simulink model "basic_cosimulation_c_1_sm_master"  (R2021b)
settings: Solver=ode4  StartTime=0.0  StopTime=inf  FixedStep=5e-05  RelTol=1e-3  EnableMultiTasking=on
PostLoadFcn:
  | %
  | % Script for validation of swtiching model design with it's respective
  | % average model.
  | %
  | % Here it is presented the design of the inverter to the 6 kW Fuel Cell
  | % model.
  | 
  | %%% Initialization %%%
  | 
  | 
  | % ------------------------------------- %
  | % ---------- Inverter Design ---------- %
  | % ------------------------------------- %
  | 
  | %%%% Nominal Parameters %%%%
  | 
  | Pnom = 50e3;                                        % Nominal Power
  | Vdc = 400;                                          % DC Voltage - Boost
  | m = 0.6;                                            % Modulation Index
  | Vnom_peak = m*Vdc/2;                                % Peak Voltage
  | Vnom_rms = Vnom_peak/sqrt(2);                       % Rms Voltage
  | FP_min = 0.9;                                       % For Reactive Power
  |                                                     % Compensation
  | Snom = Pnom/FP_min;                                 % Apparent Power
  | Irms = Pnom/(sqrt(3)*Vnom_rms);                     % Rms Curren
  | Inom_peak = Irms*sqrt(2);                           % Peak Current
  | Zbase = Vnom_peak/Inom_peak;                        % Base Impedance
  | f = 60;                                             % Nominal Frequency
  | wnom = 2*pi*60;                                     % Angular Frequency
  | 
  | % ------------------------- %
  | % Inverter LC Filter Design %
  | % ------------------------- %
  | 
  | fsw_inv = 96*60;                                    % Switching Frequency must be a multiple of the nominal frequency
  |                                                      % for proper operation of the Artemis Block
  | ripple_inv = 0.03;
  | L_inv = ((Vdc/2)-Vnom_peak)*(1/fsw_inv)/(ripple_inv*Inom_peak);
  | 
  | % - Capacitor
  | fres = 420;                                         % Filters Ressonant Frequency
  | 
  | Cf = 1/(4*L_inv*(pi^2)*(fres^2));                % Filter Capacitor
  | Rf = 1/(wnom*Cf*50);                                % Damping Resistor
  | 
  | % --- Sample Time --- %
  | 
  | Tsw = 0.00050;
  | Ts = Tsw/10;
  | 
  | % ---------------------- %
  | % Current Control Design %
  | % ---------------------- %
  | 
  | Ron = 0.001;                                        % IGBT Resistance
  | tau_i = 1e-3;                                       % Responde Time
  | kp_current = L_inv/tau_i;                           % PI Proportional Gain
  | ki_current = (Ron)/tau_i;                           % PI Integral Gain
  | 
  | decouple = (wnom*L_inv);                            % Decoupling Gain
InitFcn:
  | %
  | % Script for validation of swtiching model design with it's respective
  | % average model.
  | %
  | % Here it is presented the design of the inverter to the 6 kW Fuel Cell
  | % model.
  | 
  | %%% Initialization %%%
  | 
  | 
  | % ------------------------------------- %
  | % ---------- Inverter Design ---------- %
  | % ------------------------------------- %
  | 
  | %%%% Nominal Parameters %%%%
  | 
  | Pnom = 50e3;                                        % Nominal Power
  | Vdc = 400;                                          % DC Voltage - Boost
  | m = 0.6;                                            % Modulation Index
  | Vnom_peak = m*Vdc/2;                                % Peak Voltage
  | Vnom_rms = Vnom_peak/sqrt(2);                       % Rms Voltage
  | FP_min = 0.9;                                       % For Reactive Power
  |                                                     % Compensation
  | Snom = Pnom/FP_min;                                 % Apparent Power
  | Irms = Pnom/(sqrt(3)*Vnom_rms);                     % Rms Curren
  | Inom_peak = Irms*sqrt(2);                           % Peak Current
  | Zbase = Vnom_peak/Inom_peak;                        % Base Impedance
  | f = 60;                                             % Nominal Frequency
  | wnom = 2*pi*60;                                     % Angular Frequency
  | 
  | % ------------------------- %
  | % Inverter LC Filter Design %
  | % ------------------------- %
  | 
  | fsw_inv = 96*60;                                    % Switching Frequency must be a multiple of the nominal frequency
  |                                                      % for proper operation of the Artemis Block
  | ripple_inv = 0.03;
  | L_inv = ((Vdc/2)-Vnom_peak)*(1/fsw_inv)/(ripple_inv*Inom_peak);
  | 
  | % - Capacitor
  | fres = 420;                                         % Filters Ressonant Frequency
  | 
  | Cf = 1/(4*L_inv*(pi^2)*(fres^2));                % Filter Capacitor
  | Rf = 1/(wnom*Cf*50);                                % Damping Resistor
  | 
  | % --- Sample Time --- %
  | 
  | Tsw = 0.00050;
  | Ts = Tsw/10;
  | 
  | % ---------------------- %
  | % Current Control Design %
  | % ---------------------- %
  | 
  | Ron = 0.001;                                        % IGBT Resistance
  | tau_i = 1e-3;                                       % Responde Time
  | kp_current = L_inv/tau_i;                           % PI Proportional Gain
  | ki_current = (Ron)/tau_i;                           % PI Integral Gain
  | 
  | decouple = (wnom*L_inv);                            % Decoupling Gain
undefined symbols (not defined in the file or in its folder): D1, Delta, DiscIntNeverNeededParam, IP, j, ph, sps, UDP
libraries: spsCurrentMeasurementLib x25, spsControlledVoltageSourceLib x21, rtlab x16, spsGroundLib x13, spsThreePhaseSeriesRLCBranchLib x13, spsControlledCurrentSourceLib x11, spsVoltageMeasurementLib x10, simulink x8, rteventslib x8, powerlib_meascontrol x7, spsThreePhaseVIMeasurementLib x4, ssn_inverter_model x4
(part 2 of 5)

== system basic_cosimulation_c_1_sm_master/SM_Master/Saving RT Data1 ==
  group26 : Inport
  group27 : Inport  Port=2
  group28 : Inport  Port=3
  group29 : Inport  Port=4
  group30 : Inport  Port=5
  Bus to Vector{1..5} (5 alike) : BusToVector
  OpWriteFile26 : rtlab/DataLogging/OpWriteFile  Static_File=on  varname=data_send  Filename=data_send.mat  rtpath='./'  nrtpath='.\'  Acq_Group=26  file_size=(nls26+1)*8*(ld26/Ts)*1.5  write_offline=on  Sim_Mode=off  Nb_Samples=ld26/Ts  Buffer_size=(ld26/Ts)*8*(1+nls26)
      settings: SourceProductName=RT-LAB
  OpWriteFile27 : rtlab/DataLogging/OpWriteFile  Static_File=on  varname=data_recv  Filename=data_recv.mat  rtpath='./'  nrtpath='.\'  Acq_Group=27  file_size=(nls27+1)*8*(ld27/Ts)*1.5  write_offline=on  Sim_Mode=off  Nb_Samples=ld27/Ts  Buffer_size=(ld26/Ts)*8*(1+nls26)
      settings: SourceProductName=RT-LAB
  OpWriteFile28 : rtlab/DataLogging/OpWriteFile  Static_File=on  varname=V_injected  Filename=V_injected.mat  rtpath='./'  nrtpath='.\'  Acq_Group=28  file_size=(nls28+1)*8*(ld28/Ts)*1.5  write_offline=on  Sim_Mode=off  Nb_Samples=ld28/Ts  Buffer_size=(ld28/Ts)*8*(1+nls28)
      settings: SourceProductName=RT-LAB
  OpWriteFile29 : rtlab/DataLogging/OpWriteFile  Static_File=on  varname=Ref_V_I  Filename=Ref_V_I.mat  rtpath='./'  nrtpath='.\'  Acq_Group=29  file_size=(nls29+1)*8*(ld29/Ts)*1.5  write_offline=on  Sim_Mode=off  Nb_Samples=ld29/Ts  Buffer_size=(ld29/Ts)*8*(1+nls29)
      settings: SourceProductName=RT-LAB
  OpWriteFile30 : rtlab/DataLogging/OpWriteFile  Static_File=on  varname=PQ_ref  Filename=PQ_ref.mat  rtpath='./'  nrtpath='.\'  Acq_Group=30  file_size=(nls30+1)*8*(ld30/Ts)*1.5  write_offline=on  Sim_Mode=off  Nb_Samples=ld30/Ts  Buffer_size=(ld30/Ts)*8*(1+nls30)
      settings: SourceProductName=RT-LAB
  Terminator{1..10} (10 alike) : Terminator
  wires:
  OpWriteFile28/2 -> Terminator6/1
  OpWriteFile27/1 -> Terminator1/1
  OpWriteFile26/2 -> Terminator3/1
  OpWriteFile26/1 -> Terminator2/1
  OpWriteFile30/1 -> Terminator9/1
  OpWriteFile27/2 -> Terminator4/1
  OpWriteFile29/2 -> Terminator8/1
  OpWriteFile30/2 -> Terminator10/1
  OpWriteFile29/1 -> Terminator7/1
  OpWriteFile28/1 -> Terminator5/1
  group26/1 -> [group26]
  group27/1 -> [group27]
  group28/1 -> [group28]
  group29/1 -> [group29]
  group30/1 -> [group30]
  [group27] -> Bus to Vector1/1
  Bus to Vector1/1 -> OpWriteFile27/1
  [group29] -> Bus to Vector2/1
  Bus to Vector2/1 -> OpWriteFile29/1
  [group26] -> Bus to Vector3/1
  Bus to Vector3/1 -> OpWriteFile26/1
  [group28] -> Bus to Vector4/1
  Bus to Vector4/1 -> OpWriteFile28/1
  [group30] -> Bus to Vector5/1
  Bus to Vector5/1 -> OpWriteFile30/1

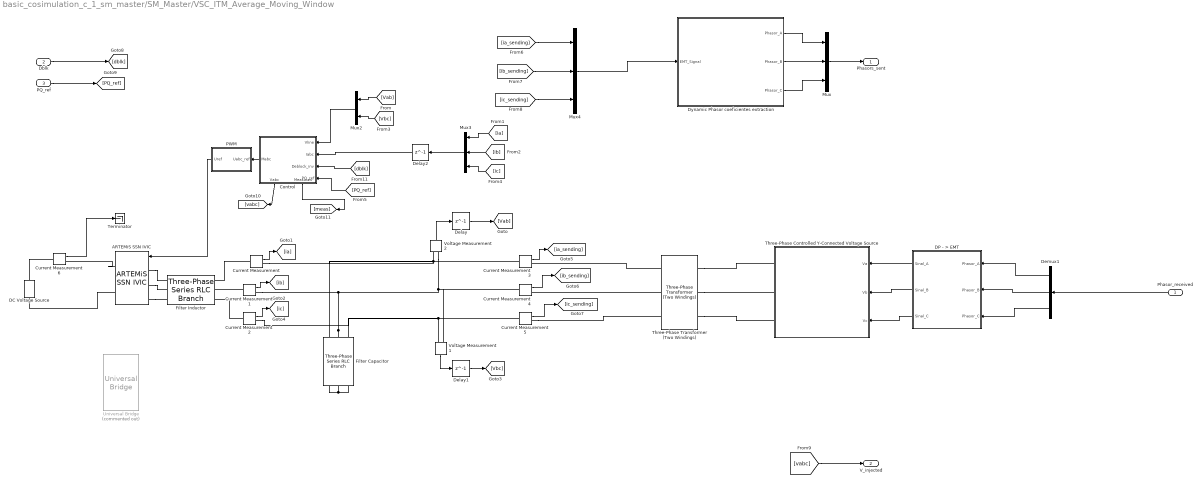
== system basic_cosimulation_c_1_sm_master/SM_Master/VSC_ITM_Average_Moving_Window ==
  Phasor_received : Inport
  Dblk : Inport  Port=2
  PQ_ref : Inport  Port=3
  ARTEMiS SSN IVIC : ssn_inverter_model/ARTEMiS SSN IVIC  Arms=3  SnubberResistance=800  SnubberCapacitance=inf  Device=IGBT / Diodes  Ron=Ron  Lon=0  ForwardVoltages=[0.001 0.001]  ForwardVoltage=0  GTOparameters=[ 10e-6 , 20e-6 ]  IGBTparameters=[ 1e-6 , 2e-6 ]*0  Measurements=None  Measurements_2=None  converterType=Rectifier
  Control : Subsystem
      settings: PortSchema="{\"entries\":[{\"content\":{\"sides\":[{\"content\":{\"connectorIds\":[\"In1\",\"In2\",\"In3\",\"In4\"]},\"type\":\"ConnectorPlacement.EquallySpacedRectSide\",\"uuid\":\"9324a1b5-9209-40a7-bba6-3b17f55cd5b4\"},{\"content\":{\"connectorIds\":[\"Out1\"],\"side\":\"RIGHT\"},\"type\":\"ConnectorPlacement.EquallySpacedRectSide\",\"uuid\":\"8b60fbd3-efee-4b93-84ca-13d5af533164\"},{\"content\":{\"connectorIds\":[],\"side\":\"TOP\"},\"type\":\"ConnectorPlacement.EquallySpacedRectSide\",\"uuid\":\"5aa46534-718a-472c-a25f-19e1867ae9eb\"},{\"content\":{\"connectorIds\":[\"Out2\",\"Out3\"],\"side\":\"BOTTOM\"},\"type\":\"ConnectorPlacement.EquallySpacedRectSide\",\"uuid\":\"4a562f23-b1c9-4bd2-8d21-c9ff01dab3f7\"},{\"content\":{\"connectorIds\":[],\"side\":\"HIDDEN\"},\"type\":\"ConnectorPlacement.EquallySpacedRectSide\",\"uuid\":\"2bae700d-a0ed-419d-b89d-d5ddfcfc4dca\"}]},\"type\":\"ConnectorPlacement.EquallySpacedConnector\",\"uuid\":\"0ed67f90-7cb8-4c5b-bc99-423fd2f61638\"}],\"packageUris\":[\"http://schema.mathworks.com/mf0/Connector/R2020b\"],\"version\":\"1.0\"}"
  Current Measurement{,1..6} (7 alike) : spsCurrentMeasurementLib/Current Measurement  PhasorSimulation=off  OutputType=Complex  PSBequivalent=0
  DC Voltage Source : spsDCVoltageSourceLib/DC Voltage Source  Amplitude=Vdc  Measurements=None
  DP - > EMT : Subsystem
  Delay : Delay  DelayLength=1
  Delay1 : Delay  DelayLength=1
  Delay2 : Delay  DelayLength=1
  Demux1 : Demux  Outputs=3
  Dynamic Phasor coeficientes extraction : Subsystem
  Filter Capacitor : spsThreePhaseSeriesRLCBranchLib/Three-Phase Series RLC Branch  LConnTagsString=A|B|C  RConnTagsString=A|B|C  BranchType=RC  Resistance=Rf  Inductance=L_inv  Capacitance=Cf  Measurements=None
  Filter Inductor : spsThreePhaseSeriesRLCBranchLib/Three-Phase Series RLC Branch  LConnTagsString=A|B|C  RConnTagsString=A|B|C  BranchType=RL  Resistance=1e-3  Inductance=L_inv  Capacitance=1e-6  Measurements=None
  Mux : Mux  Inputs=3
  Mux2 : Mux  Inputs=2
  Mux3 : Mux  Inputs=3
  Mux4 : Mux  Inputs=3
  PWM : Subsystem  AncestorBlock=LafaeLib/PV System/PV System Detailed/VSC_Control/PWM
  Terminator : Terminator
  Three-Phase Transformer (Two Windings) : spsThreePhaseTransformerTwoWindingsLib/Three-Phase Transformer (Two Windings)  Winding1Connection=Delta (D1)  Winding2Connection=Yg  CoreType=Three single-phase transformers  SetSaturation=off  Hysteresis=off  DataFile='hysteresis'  SetInitialFlux=off  Measurements=None  UNITS=pu  NominalPower=[ 80e3 , 60 ]  Winding1=[ Vnom_rms*sqrt(3) , 0.002 , 0.08 ]  Winding2=[440 , 0.002 , 0.02 ]  Rm=500  Lm=500  L0=0.5  Saturation=[ 0,0 ; 0.0024,1.2 ; 1.0,1.52 ]  InitialFluxes=[ 0.8 , -0.8 , 0.7 ]  BreakLoop=off  DiscreteSolver=Trapezoidal iterative  DataType=off  TransfoNumber=1
  "Three-Phase Controlled Y-Connected Voltage Source " : Subsystem
  Universal Bridge : spsUniversalBridgeLib/Universal Bridge  Commented=on  Arms=3  SnubberResistance=1e5  SnubberCapacitance=inf  Device=Average-model based VSC  Ron=1e-3  Lon=0  ForwardVoltages="[  0  0  ]"  ForwardVoltage=0  GTOparameters=[ 10e-6 , 20e-6 ]  IGBTparameters=[ 1e-6 , 2e-6 ]  Measurements=None  Measurements_2=None  converterType=Rectifier
  Voltage Measurement1 : spsVoltageMeasurementLib/Voltage Measurement  PhasorSimulation=off  OutputType=Complex  PSBequivalent=0
  Voltage Measurement2 : spsVoltageMeasurementLib/Voltage Measurement  PhasorSimulation=off  OutputType=Complex  PSBequivalent=0
  Phasors_sent : Outport
  V_injected : Outport  Port=2
  wires:
  DP - > EMT/1(Sinal_A) -> "Three-Phase Controlled Y-Connected Voltage Source "/1(Va)
  DP - > EMT/2(Sinal_B) -> "Three-Phase Controlled Y-Connected Voltage Source "/2(Vb)
  Mux3/1 -> Delay2/1
  [PQ_ref] -> Control/4(PQ_ref)
  Delay2/1 -> Control/2(Iabc)
  [dblk] -> Control/3(Deblock_inv)
  Delay/1 -> [Vab]
  [ic] -> Mux3/3
  Voltage Measurement1/1 -> Delay1/1
  [Vab] -> Mux2/1
  [ib] -> Mux3/2
  Voltage Measurement2/1 -> Delay/1
  [ia] -> Mux3/1
  Current Measurement/1 -> [ia]
  Delay1/1 -> [Vbc]
  Mux2/1 -> Control/1(Vline)
  Current Measurement1/1 -> [ib]
  Control/2(Measures) -> [meas]
  [Vbc] -> Mux2/2
  Current Measurement2/1 -> [ic]
  Current Measurement5/1 -> [ic_sending]
  Current Measurement4/1 -> [ib_sending]
  Current Measurement3/1 -> [ia_sending]
  Mux4/1 -> Dynamic Phasor coeficientes extraction/1(EMT_Signal)
  [vabc] -> V_injected/1
  Dblk/1 -> [dblk]
  PQ_ref/1 -> [PQ_ref]
  Control/3(Vabc) -> [vabc]
  [ia_sending] -> Mux4/1
  [ib_sending] -> Mux4/2
  [ic_sending] -> Mux4/3
  Control/1(Mabc) -> PWM/1(Uabc_ref)
  DP - > EMT/3(Sinal_C) -> "Three-Phase Controlled Y-Connected Voltage Source "/3(Vc)
  Current Measurement6/1 -> Terminator/1
  PWM/1(Uref) -> ARTEMiS SSN IVIC/1
  Dynamic Phasor coeficientes extraction/1(Phasor_A) -> Mux/1
  Dynamic Phasor coeficientes extraction/3(Phasor_C) -> Mux/3
  Demux1/2 -> DP - > EMT/2(Phasor_B)
  Dynamic Phasor coeficientes extraction/2(Phasor_B) -> Mux/2
  Phasor_received/1 -> Demux1/1
  Demux1/3 -> DP - > EMT/3(Phasor_C)
  Demux1/1 -> DP - > EMT/1(Phasor_A)
  Mux/1 -> Phasors_sent/1
  connections:
  Filter Capacitor/LConn2 -- Current Measurement1/RConn1 -- Voltage Measurement1/LConn1 -- Current Measurement4/LConn1 -- Voltage Measurement2/LConn2
  Filter Capacitor/RConn2 -- Filter Capacitor/RConn3 -- Filter Capacitor/RConn1
  DC Voltage Source/RConn1 -- Current Measurement6/LConn1
  Current Measurement3/LConn1 -- Voltage Measurement2/LConn1 -- Filter Capacitor/LConn1 -- Current Measurement/RConn1
  Current Measurement5/LConn1 -- Voltage Measurement1/LConn2 -- Filter Capacitor/LConn3 -- Current Measurement2/RConn1
  Current Measurement2/LConn1 -- Filter Inductor/RConn3
  Current Measurement/LConn1 -- Filter Inductor/RConn1
  Current Measurement1/LConn1 -- Filter Inductor/RConn2
  ARTEMiS SSN IVIC/LConn1 -- Filter Inductor/LConn1
  ARTEMiS SSN IVIC/LConn2 -- Filter Inductor/LConn2
  ARTEMiS SSN IVIC/LConn3 -- Filter Inductor/LConn3
  ARTEMiS SSN IVIC/RConn1 -- Current Measurement6/RConn1
  ARTEMiS SSN IVIC/RConn2 -- DC Voltage Source/LConn1
  Three-Phase Transformer (Two Windings)/RConn1 -- "Three-Phase Controlled Y-Connected Voltage Source "/RConn1
  Three-Phase Transformer (Two Windings)/RConn2 -- "Three-Phase Controlled Y-Connected Voltage Source "/RConn2
  Three-Phase Transformer (Two Windings)/RConn3 -- "Three-Phase Controlled Y-Connected Voltage Source "/RConn3
  Three-Phase Transformer (Two Windings)/LConn1 -- Current Measurement3/RConn1
  Three-Phase Transformer (Two Windings)/LConn2 -- Current Measurement4/RConn1
  Current Measurement5/RConn1 -- Three-Phase Transformer (Two Windings)/LConn3

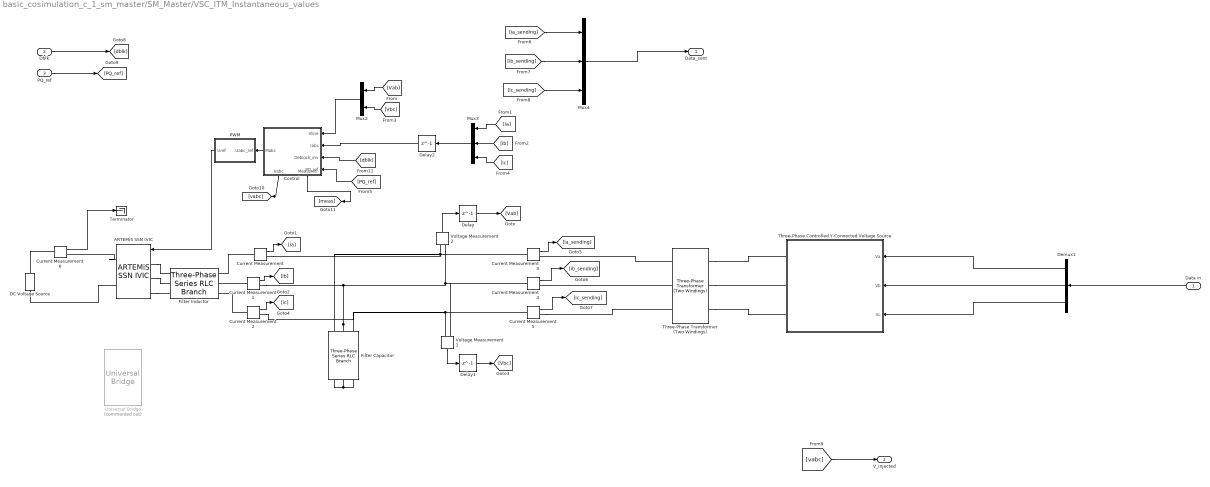
== system basic_cosimulation_c_1_sm_master/SM_Master/VSC_ITM_Instantaneous_values ==
  Data in : Inport
  Dblk : Inport  Port=2
  PQ_ref : Inport  Port=3
  ARTEMiS SSN IVIC : ssn_inverter_model/ARTEMiS SSN IVIC  Arms=3  SnubberResistance=800  SnubberCapacitance=inf  Device=IGBT / Diodes  Ron=Ron  Lon=0  ForwardVoltages=[0.001 0.001]  ForwardVoltage=0  GTOparameters=[ 10e-6 , 20e-6 ]  IGBTparameters=[ 1e-6 , 2e-6 ]*0  Measurements=None  Measurements_2=None  converterType=Rectifier
  Control : Subsystem
      settings: PortSchema="{\"entries\":[{\"content\":{\"sides\":[{\"content\":{\"connectorIds\":[\"In1\",\"In2\",\"In3\",\"In4\"]},\"type\":\"ConnectorPlacement.EquallySpacedRectSide\",\"uuid\":\"9324a1b5-9209-40a7-bba6-3b17f55cd5b4\"},{\"content\":{\"connectorIds\":[\"Out1\"],\"side\":\"RIGHT\"},\"type\":\"ConnectorPlacement.EquallySpacedRectSide\",\"uuid\":\"8b60fbd3-efee-4b93-84ca-13d5af533164\"},{\"content\":{\"connectorIds\":[],\"side\":\"TOP\"},\"type\":\"ConnectorPlacement.EquallySpacedRectSide\",\"uuid\":\"5aa46534-718a-472c-a25f-19e1867ae9eb\"},{\"content\":{\"connectorIds\":[\"Out2\",\"Out3\"],\"side\":\"BOTTOM\"},\"type\":\"ConnectorPlacement.EquallySpacedRectSide\",\"uuid\":\"4a562f23-b1c9-4bd2-8d21-c9ff01dab3f7\"},{\"content\":{\"connectorIds\":[],\"side\":\"HIDDEN\"},\"type\":\"ConnectorPlacement.EquallySpacedRectSide\",\"uuid\":\"2bae700d-a0ed-419d-b89d-d5ddfcfc4dca\"}]},\"type\":\"ConnectorPlacement.EquallySpacedConnector\",\"uuid\":\"0ed67f90-7cb8-4c5b-bc99-423fd2f61638\"}],\"packageUris\":[\"http://schema.mathworks.com/mf0/Connector/R2020b\"],\"version\":\"1.0\"}"
  Current Measurement{,1..6} (7 alike) : spsCurrentMeasurementLib/Current Measurement  PhasorSimulation=off  OutputType=Complex  PSBequivalent=0
  DC Voltage Source : spsDCVoltageSourceLib/DC Voltage Source  Amplitude=Vdc  Measurements=None
  Delay : Delay  DelayLength=1
  Delay1 : Delay  DelayLength=1
  Delay2 : Delay  DelayLength=1
  Demux1 : Demux  Outputs=3
  Filter Capacitor : spsThreePhaseSeriesRLCBranchLib/Three-Phase Series RLC Branch  LConnTagsString=A|B|C  RConnTagsString=A|B|C  BranchType=RC  Resistance=Rf  Inductance=L_inv  Capacitance=Cf  Measurements=None
  Filter Inductor : spsThreePhaseSeriesRLCBranchLib/Three-Phase Series RLC Branch  LConnTagsString=A|B|C  RConnTagsString=A|B|C  BranchType=RL  Resistance=1e-3  Inductance=L_inv  Capacitance=1e-6  Measurements=None
  Mux2 : Mux  Inputs=2
  Mux3 : Mux  Inputs=3
  Mux4 : Mux  Inputs=3
  PWM : Subsystem  AncestorBlock=LafaeLib/PV System/PV System Detailed/VSC_Control/PWM
  Terminator : Terminator
  Three-Phase Transformer (Two Windings) : spsThreePhaseTransformerTwoWindingsLib/Three-Phase Transformer (Two Windings)  Winding1Connection=Delta (D1)  Winding2Connection=Yg  CoreType=Three single-phase transformers  SetSaturation=off  Hysteresis=off  DataFile='hysteresis'  SetInitialFlux=off  Measurements=None  UNITS=pu  NominalPower=[ 80e3 , 60 ]  Winding1=[ Vnom_rms*sqrt(3) , 0.002 , 0.08 ]  Winding2=[440 , 0.002 , 0.02 ]  Rm=500  Lm=500  L0=0.5  Saturation=[ 0,0 ; 0.0024,1.2 ; 1.0,1.52 ]  InitialFluxes=[ 0.8 , -0.8 , 0.7 ]  BreakLoop=off  DiscreteSolver=Trapezoidal iterative  DataType=off  TransfoNumber=1
  "Three-Phase Controlled Y-Connected Voltage Source " : Subsystem
  Universal Bridge : spsUniversalBridgeLib/Universal Bridge  Commented=on  Arms=3  SnubberResistance=1e5  SnubberCapacitance=inf  Device=Average-model based VSC  Ron=1e-3  Lon=0  ForwardVoltages="[  0  0  ]"  ForwardVoltage=0  GTOparameters=[ 10e-6 , 20e-6 ]  IGBTparameters=[ 1e-6 , 2e-6 ]  Measurements=None  Measurements_2=None  converterType=Rectifier
  Voltage Measurement1 : spsVoltageMeasurementLib/Voltage Measurement  PhasorSimulation=off  OutputType=Complex  PSBequivalent=0
  Voltage Measurement2 : spsVoltageMeasurementLib/Voltage Measurement  PhasorSimulation=off  OutputType=Complex  PSBequivalent=0
  Data_sent : Outport
  V_injected : Outport  Port=2
  wires:
  Demux1/1 -> "Three-Phase Controlled Y-Connected Voltage Source "/1(Va)
  Demux1/2 -> "Three-Phase Controlled Y-Connected Voltage Source "/2(Vb)
  Mux3/1 -> Delay2/1
  [PQ_ref] -> Control/4(PQ_ref)
  Delay2/1 -> Control/2(Iabc)
  [dblk] -> Control/3(Deblock_inv)
  Delay/1 -> [Vab]
  [ic] -> Mux3/3
  Voltage Measurement1/1 -> Delay1/1
  [Vab] -> Mux2/1
  [ib] -> Mux3/2
  Voltage Measurement2/1 -> Delay/1
  [ia] -> Mux3/1
  Current Measurement/1 -> [ia]
  Delay1/1 -> [Vbc]
  Mux2/1 -> Control/1(Vline)
  Current Measurement1/1 -> [ib]
  Control/2(Measures) -> [meas]
  [Vbc] -> Mux2/2
  Current Measurement2/1 -> [ic]
  Current Measurement5/1 -> [ic_sending]
  Current Measurement4/1 -> [ib_sending]
  Current Measurement3/1 -> [ia_sending]
  Mux4/1 -> Data_sent/1
  [vabc] -> V_injected/1
  Dblk/1 -> [dblk]
  PQ_ref/1 -> [PQ_ref]
  Control/3(Vabc) -> [vabc]
  [ia_sending] -> Mux4/1
  [ib_sending] -> Mux4/2
  [ic_sending] -> Mux4/3
  Control/1(Mabc) -> PWM/1(Uabc_ref)
  Demux1/3 -> "Three-Phase Controlled Y-Connected Voltage Source "/3(Vc)
  Current Measurement6/1 -> Terminator/1
  PWM/1(Uref) -> ARTEMiS SSN IVIC/1
  Data in/1 -> Demux1/1
  connections:
  Filter Capacitor/LConn2 -- Current Measurement1/RConn1 -- Voltage Measurement1/LConn1 -- Current Measurement4/LConn1 -- Voltage Measurement2/LConn2
  Filter Capacitor/RConn2 -- Filter Capacitor/RConn3 -- Filter Capacitor/RConn1
  DC Voltage Source/RConn1 -- Current Measurement6/LConn1
  Current Measurement3/LConn1 -- Voltage Measurement2/LConn1 -- Filter Capacitor/LConn1 -- Current Measurement/RConn1
  Current Measurement5/LConn1 -- Voltage Measurement1/LConn2 -- Filter Capacitor/LConn3 -- Current Measurement2/RConn1
  Current Measurement2/LConn1 -- Filter Inductor/RConn3
  Current Measurement/LConn1 -- Filter Inductor/RConn1
  Current Measurement1/LConn1 -- Filter Inductor/RConn2
  ARTEMiS SSN IVIC/LConn1 -- Filter Inductor/LConn1
  ARTEMiS SSN IVIC/LConn2 -- Filter Inductor/LConn2
  ARTEMiS SSN IVIC/LConn3 -- Filter Inductor/LConn3
  ARTEMiS SSN IVIC/RConn1 -- Current Measurement6/RConn1
  ARTEMiS SSN IVIC/RConn2 -- DC Voltage Source/LConn1
  Three-Phase Transformer (Two Windings)/RConn1 -- "Three-Phase Controlled Y-Connected Voltage Source "/RConn1
  Three-Phase Transformer (Two Windings)/RConn2 -- "Three-Phase Controlled Y-Connected Voltage Source "/RConn2
  Three-Phase Transformer (Two Windings)/RConn3 -- "Three-Phase Controlled Y-Connected Voltage Source "/RConn3
  Three-Phase Transformer (Two Windings)/LConn1 -- Current Measurement3/RConn1
  Three-Phase Transformer (Two Windings)/LConn2 -- Current Measurement4/RConn1
  Current Measurement5/RConn1 -- Three-Phase Transformer (Two Windings)/LConn3

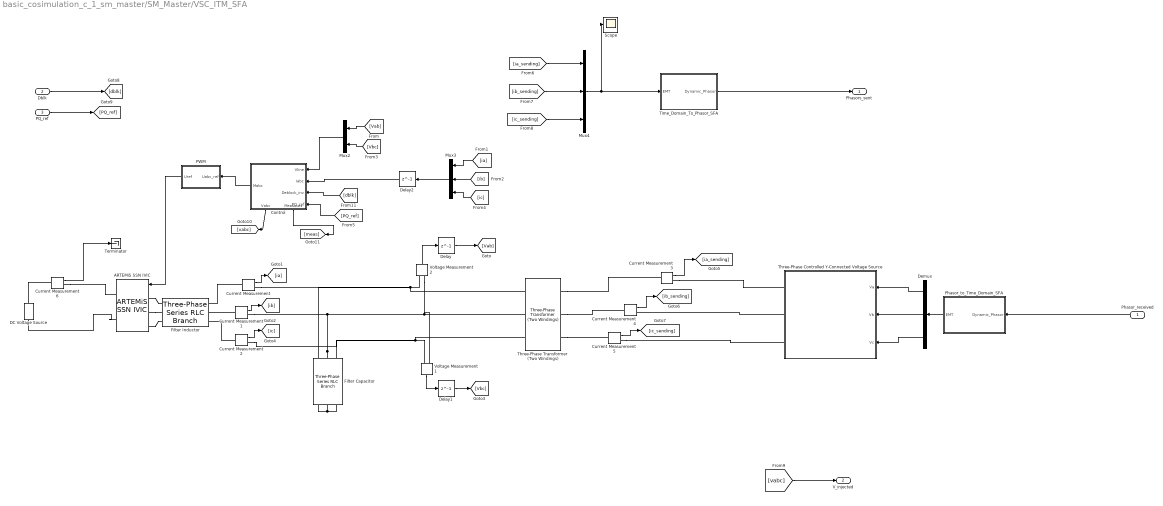
== system basic_cosimulation_c_1_sm_master/SM_Master/VSC_ITM_SFA ==
  Phasor_received : Inport
  Dblk : Inport  Port=2
  PQ_ref : Inport  Port=3
  ARTEMiS SSN IVIC : ssn_inverter_model/ARTEMiS SSN IVIC  Arms=3  SnubberResistance=800  SnubberCapacitance=inf  Device=IGBT / Diodes  Ron=Ron  Lon=0  ForwardVoltages=[0.001 0.001]  ForwardVoltage=0  GTOparameters=[ 10e-6 , 20e-6 ]  IGBTparameters=[ 1e-6 , 2e-6 ]*0  Measurements=None  Measurements_2=None  converterType=Rectifier
  Control : Subsystem
      settings: PortSchema="{\"entries\":[{\"content\":{\"sides\":[{\"content\":{\"connectorIds\":[\"In1\",\"In2\",\"In3\",\"In4\"]},\"type\":\"ConnectorPlacement.EquallySpacedRectSide\",\"uuid\":\"9324a1b5-9209-40a7-bba6-3b17f55cd5b4\"},{\"content\":{\"connectorIds\":[\"Out1\"],\"side\":\"RIGHT\"},\"type\":\"ConnectorPlacement.EquallySpacedRectSide\",\"uuid\":\"8b60fbd3-efee-4b93-84ca-13d5af533164\"},{\"content\":{\"connectorIds\":[],\"side\":\"TOP\"},\"type\":\"ConnectorPlacement.EquallySpacedRectSide\",\"uuid\":\"5aa46534-718a-472c-a25f-19e1867ae9eb\"},{\"content\":{\"connectorIds\":[\"Out2\",\"Out3\"],\"side\":\"BOTTOM\"},\"type\":\"ConnectorPlacement.EquallySpacedRectSide\",\"uuid\":\"4a562f23-b1c9-4bd2-8d21-c9ff01dab3f7\"},{\"content\":{\"connectorIds\":[],\"side\":\"HIDDEN\"},\"type\":\"ConnectorPlacement.EquallySpacedRectSide\",\"uuid\":\"2bae700d-a0ed-419d-b89d-d5ddfcfc4dca\"}]},\"type\":\"ConnectorPlacement.EquallySpacedConnector\",\"uuid\":\"0ed67f90-7cb8-4c5b-bc99-423fd2f61638\"}],\"packageUris\":[\"http://schema.mathworks.com/mf0/Connector/R2020b\"],\"version\":\"1.0\"}"
  Current Measurement{,1..6} (7 alike) : spsCurrentMeasurementLib/Current Measurement  PhasorSimulation=off  OutputType=Complex  PSBequivalent=0
  DC Voltage Source : spsDCVoltageSourceLib/DC Voltage Source  Amplitude=Vdc  Measurements=None
  Delay : Delay  DelayLength=1
  Delay1 : Delay  DelayLength=1
  Delay2 : Delay  DelayLength=1
  Demux : Demux  Outputs=3
  Filter Capacitor : spsThreePhaseSeriesRLCBranchLib/Three-Phase Series RLC Branch  LConnTagsString=A|B|C  RConnTagsString=A|B|C  BranchType=RC  Resistance=Rf  Inductance=L_inv  Capacitance=Cf  Measurements=None
  Filter Inductor : spsThreePhaseSeriesRLCBranchLib/Three-Phase Series RLC Branch  LConnTagsString=A|B|C  RConnTagsString=A|B|C  BranchType=RL  Resistance=1e-3  Inductance=L_inv  Capacitance=1e-6  Measurements=None
  Mux2 : Mux  Inputs=2
  Mux3 : Mux  Inputs=3
  Mux4 : Mux  Inputs=3
  PWM : Subsystem  AncestorBlock=LafaeLib/PV System/PV System Detailed/VSC_Control/PWM
  Phasor_to_Time_Domain_SFA : Subsystem  mask(Time domain from Dynamic Phasor){offset=60}
      mask prompts: offset "Frequency shift"
      mask help: This block extracts Time Domain Signals from the Dynamic Phasor by using the SFA method. It is usable only for three-phase signals
  Scope : Scope
  Terminator : Terminator
  Three-Phase Transformer (Two Windings) : spsThreePhaseTransformerTwoWindingsLib/Three-Phase Transformer (Two Windings)  Winding1Connection=Delta (D1)  Winding2Connection=Yg  CoreType=Three single-phase transformers  SetSaturation=off  Hysteresis=off  DataFile='hysteresis'  SetInitialFlux=off  Measurements=None  UNITS=pu  NominalPower=[ 80e3 , 60 ]  Winding1=[ Vnom_rms*sqrt(3) , 0.002 , 0.08 ]  Winding2=[440 , 0.002 , 0.02 ]  Rm=500  Lm=500  L0=0.5  Saturation=[ 0,0 ; 0.0024,1.2 ; 1.0,1.52 ]  InitialFluxes=[ 0.8 , -0.8 , 0.7 ]  BreakLoop=off  DiscreteSolver=Trapezoidal iterative  DataType=off  TransfoNumber=1
  "Three-Phase Controlled Y-Connected Voltage Source " : Subsystem
  Time_Domain_To_Phasor_SFA : Subsystem  mask(SFA){offset=60}
      mask prompts: offset "Frequency shift"
      mask help: This block extracts Dynamic Phasor by using the SFA method. It is usable only for three-phase signals
  Voltage Measurement1 : spsVoltageMeasurementLib/Voltage Measurement  PhasorSimulation=off  OutputType=Complex  PSBequivalent=0
  Voltage Measurement2 : spsVoltageMeasurementLib/Voltage Measurement  PhasorSimulation=off  OutputType=Complex  PSBequivalent=0
  Phasors_sent : Outport
  V_injected : Outport  Port=2
  wires:
  Demux/1 -> "Three-Phase Controlled Y-Connected Voltage Source "/1(Va)
  Demux/2 -> "Three-Phase Controlled Y-Connected Voltage Source "/2(Vb)
  Mux3/1 -> Delay2/1
  [PQ_ref] -> Control/4(PQ_ref)
  Delay2/1 -> Control/2(Iabc)
  [dblk] -> Control/3(Deblock_inv)
  Delay/1 -> [Vab]
  [ic] -> Mux3/3
  Voltage Measurement1/1 -> Delay1/1
  [Vab] -> Mux2/1
  [ib] -> Mux3/2
  Voltage Measurement2/1 -> Delay/1
  [ia] -> Mux3/1
  Current Measurement/1 -> [ia]
  Delay1/1 -> [Vbc]
  Mux2/1 -> Control/1(Vline)
  Current Measurement1/1 -> [ib]
  Control/2(Measures) -> [meas]
  [Vbc] -> Mux2/2
  Current Measurement2/1 -> [ic]
  [vabc] -> V_injected/1
  Dblk/1 -> [dblk]
  PQ_ref/1 -> [PQ_ref]
  Control/3(Vabc) -> [vabc]
  [ia_sending] -> Mux4/1
  [ib_sending] -> Mux4/2
  [ic_sending] -> Mux4/3
  Control/1(Mabc) -> PWM/1(Uabc_ref)
  Demux/3 -> "Three-Phase Controlled Y-Connected Voltage Source "/3(Vc)
  Current Measurement6/1 -> Terminator/1
  Current Measurement4/1 -> [ib_sending]
  Current Measurement5/1 -> [ic_sending]
  Current Measurement3/1 -> [ia_sending]
  Phasor_received/1 -> Phasor_to_Time_Domain_SFA/1(Dynamic_Phasor)
  Time_Domain_To_Phasor_SFA/1(Dynamic_Phasor) -> Phasors_sent/1
  Mux4/1 -> Time_Domain_To_Phasor_SFA/1(EMT), Scope/1
  PWM/1(Uref) -> ARTEMiS SSN IVIC/1
  Phasor_to_Time_Domain_SFA/1(EMT) -> Demux/1
  connections:
  Filter Capacitor/RConn2 -- Filter Capacitor/RConn3 -- Filter Capacitor/RConn1
  DC Voltage Source/RConn1 -- Current Measurement6/LConn1
  Current Measurement2/LConn1 -- Filter Inductor/RConn3
  Current Measurement/LConn1 -- Filter Inductor/RConn1
  Current Measurement1/LConn1 -- Filter Inductor/RConn2
  ARTEMiS SSN IVIC/LConn1 -- Filter Inductor/LConn1
  ARTEMiS SSN IVIC/LConn2 -- Filter Inductor/LConn2
  ARTEMiS SSN IVIC/LConn3 -- Filter Inductor/LConn3
  Current Measurement6/RConn1 -- ARTEMiS SSN IVIC/RConn1
  ARTEMiS SSN IVIC/RConn2 -- DC Voltage Source/LConn1
  Filter Capacitor/LConn1 -- Current Measurement/RConn1 -- Three-Phase Transformer (Two Windings)/LConn1 -- Voltage Measurement2/LConn1
  Filter Capacitor/LConn3 -- Current Measurement2/RConn1 -- Three-Phase Transformer (Two Windings)/LConn3 -- Voltage Measurement1/LConn2
  Filter Capacitor/LConn2 -- Three-Phase Transformer (Two Windings)/LConn2 -- Voltage Measurement1/LConn1 -- Voltage Measurement2/LConn2 -- Current Measurement1/RConn1
  "Three-Phase Controlled Y-Connected Voltage Source "/RConn2 -- Current Measurement4/RConn1
  Current Measurement3/RConn1 -- "Three-Phase Controlled Y-Connected Voltage Source "/RConn1
  Current Measurement5/RConn1 -- "Three-Phase Controlled Y-Connected Voltage Source "/RConn3
  Three-Phase Transformer (Two Windings)/RConn2 -- Current Measurement4/LConn1
  Three-Phase Transformer (Two Windings)/RConn3 -- Current Measurement5/LConn1
  Three-Phase Transformer (Two Windings)/RConn1 -- Current Measurement3/LConn1

== system basic_cosimulation_c_1_sm_master/SM_Master/rtlab_send_subsystem ==
  Subsystem1 : Subsystem
  wires:
  [rtlab_send_1] -> Subsystem1/1(In1)
  [rtlab_send_2] -> Subsystem1/2(In2)
  [rtlab_send_3] -> Subsystem1/3(In3)
  [rtlab_send_4] -> Subsystem1/4(In4)
  [rtlab_send_5] -> Subsystem1/5(In5)

== system basic_cosimulation_c_1_sm_master/SM_Master/Circuit_ITM_Source/Controllable Voltage Source 1 ==
  Amplitude [V] : Inport
  Phase [Deg] : Inport  Port=2
  Frequency [Hz] : Inport  Port=3
  Constant1 : Constant  Value=2*pi/3
  Controlled Voltage Source3 : spsControlledVoltageSourceLib/Controlled Voltage Source  Initialize=on  Source_Type=AC  Amplitude=0  Phase=0  Frequency=0  Measurements=None
  Controlled Voltage Source4 : spsControlledVoltageSourceLib/Controlled Voltage Source  Initialize=on  Source_Type=AC  Amplitude=0  Phase=0  Frequency=0  Measurements=None
  Controlled Voltage Source5 : spsControlledVoltageSourceLib/Controlled Voltage Source  Initialize=on  Source_Type=AC  Amplitude=0  Phase=0  Frequency=0  Measurements=None
  Cos : Trigonometry  Operator=cos
  Cos1 : Trigonometry  Operator=cos
  Cos2 : Trigonometry  Operator=cos
  Gain : Gain  Gain=2*pi
  Gain1 : Gain  Gain=pi/180
  Ground5 : spsGroundLib/Ground  LConnTagsString=a
  Integrator : Integrator  WrapState=on  WrappedStateUpperValue=2*pi  WrappedStateLowerValue=0
  Product : Product
  Product1 : Product
  Product2 : Product
  Sum : Sum  Inputs=++-
  Sum1 : Sum  Inputs=+++
  Sum2 : Sum  Inputs=|++
  A : PMIOPort  Side=Right
  B : PMIOPort  Port=2  Side=Right
  C : PMIOPort  Port=3  Side=Right
  wires:
  Sum/1 -> Cos1/1
  Amplitude [V]/1 -> Product2/1, Product1/1, Product/1
  Integrator/1 -> [phase]
  Gain/1 -> Integrator/1
  Phase [Deg]/1 -> Gain1/1
  Constant1/1 -> Sum/3, Sum1/2
  Sum2/1 -> Cos/1
  Product/1 -> Controlled Voltage Source3/1
  Cos/1 -> Product/2
  [phase] -> Sum2/1, Sum/2, Sum1/1
  Product1/1 -> Controlled Voltage Source4/1
  Product2/1 -> Controlled Voltage Source5/1
  Sum1/1 -> Cos2/1
  Cos1/1 -> Product1/2
  Cos2/1 -> Product2/2
  Frequency [Hz]/1 -> [freq_ref], Gain/1
  Gain1/1 -> Sum1/3, Sum/1, Sum2/2
  connections:
  Controlled Voltage Source4/RConn1 -- B/RConn1
  Controlled Voltage Source3/RConn1 -- A/RConn1
  Controlled Voltage Source5/RConn1 -- C/RConn1
  Controlled Voltage Source4/LConn1 -- Ground5/LConn1 -- Controlled Voltage Source5/LConn1 -- Controlled Voltage Source3/LConn1

== system basic_cosimulation_c_1_sm_master/SM_Master/Circuit_ITM_Source/Three-Phase Controlled Y-Connected Current Source ==
  Ia : Inport
  Ib : Inport  Port=2
  Ic : Inport  Port=3
  Controlled Current Source : spsControlledCurrentSourceLib/Controlled Current Source  Initialize=on  Source_Type=AC  Amplitude=0  Phase=0  Frequency=0  Measurements=None
  Controlled Current Source1 : spsControlledCurrentSourceLib/Controlled Current Source  Initialize=on  Source_Type=AC  Amplitude=0  Phase=0  Frequency=0  Measurements=None
  Controlled Current Source2 : spsControlledCurrentSourceLib/Controlled Current Source  Initialize=on  Source_Type=AC  Amplitude=0  Phase=0  Frequency=0  Measurements=None
  Ground1 : spsGroundLib/Ground  LConnTagsString=a
  A : PMIOPort  Side=Left
  B : PMIOPort  Port=2  Side=Left
  C : PMIOPort  Port=3  Side=Left
  wires:
  Ia/1 -> Controlled Current Source/1
  Ic/1 -> Controlled Current Source2/1
  Ib/1 -> Controlled Current Source1/1
  connections:
  Controlled Current Source/RConn1 -- Controlled Current Source2/RConn1 -- Ground1/LConn1 -- Controlled Current Source1/RConn1
  C/RConn1 -- Controlled Current Source2/LConn1
  B/RConn1 -- Controlled Current Source1/LConn1
  Controlled Current Source/LConn1 -- A/RConn1

== system basic_cosimulation_c_1_sm_master/SM_Master/Circuit_ITM_Source_DP_AW/Controllable Voltage Source  ==
  Amplitude [V] : Inport
  Phase [Deg] : Inport  Port=2
  Frequency [Hz] : Inport  Port=3
  Constant1 : Constant  Value=2*pi/3
  Controlled Voltage Source3 : spsControlledVoltageSourceLib/Controlled Voltage Source  Initialize=on  Source_Type=AC  Amplitude=0  Phase=0  Frequency=0  Measurements=None
  Controlled Voltage Source4 : spsControlledVoltageSourceLib/Controlled Voltage Source  Initialize=on  Source_Type=AC  Amplitude=0  Phase=0  Frequency=0  Measurements=None
  Controlled Voltage Source5 : spsControlledVoltageSourceLib/Controlled Voltage Source  Initialize=on  Source_Type=AC  Amplitude=0  Phase=0  Frequency=0  Measurements=None
  Cos : Trigonometry  Operator=cos
  Cos1 : Trigonometry  Operator=cos
  Cos2 : Trigonometry  Operator=cos
  Gain : Gain  Gain=2*pi
  Gain1 : Gain  Gain=pi/180
  Ground5 : spsGroundLib/Ground  LConnTagsString=a
  Integrator : Integrator  WrapState=on  WrappedStateUpperValue=2*pi  WrappedStateLowerValue=0
  Product : Product
  Product1 : Product
  Product2 : Product
  Sum : Sum  Inputs=++-
  Sum1 : Sum  Inputs=+++
  Sum2 : Sum  Inputs=|++
  A : PMIOPort  Side=Right
  B : PMIOPort  Port=2  Side=Right
  C : PMIOPort  Port=3  Side=Right
  wires:
  Sum/1 -> Cos1/1
  Amplitude [V]/1 -> Product2/1, Product1/1, Product/1
  Integrator/1 -> [phase]
  Gain/1 -> Integrator/1
  Phase [Deg]/1 -> Gain1/1
  Constant1/1 -> Sum/3, Sum1/2
  Sum2/1 -> Cos/1
  Product/1 -> Controlled Voltage Source3/1
  Cos/1 -> Product/2
  [phase] -> Sum2/1, Sum/2, Sum1/1
  Product1/1 -> Controlled Voltage Source4/1
  Product2/1 -> Controlled Voltage Source5/1
  Sum1/1 -> Cos2/1
  Cos1/1 -> Product1/2
  Cos2/1 -> Product2/2
  Frequency [Hz]/1 -> [freq_ref], Gain/1
  Gain1/1 -> Sum1/3, Sum/1, Sum2/2
  connections:
  Controlled Voltage Source4/RConn1 -- B/RConn1
  Controlled Voltage Source3/RConn1 -- A/RConn1
  Controlled Voltage Source5/RConn1 -- C/RConn1
  Controlled Voltage Source4/LConn1 -- Ground5/LConn1 -- Controlled Voltage Source5/LConn1 -- Controlled Voltage Source3/LConn1

== system basic_cosimulation_c_1_sm_master/SM_Master/Circuit_ITM_Source_DP_AW/DP - > EMT ==
  Phasor_A : Inport
  Phasor_B : Inport  Port=2
  Phasor_C : Inport  Port=3
  Demux : Demux  Outputs=2
  Demux1 : Demux  Outputs=2
  Demux2 : Demux  Outputs=2
  Subsystem : Subsystem
  Subsystem1 : Subsystem
  Subsystem2 : Subsystem
  Sinal_A : Outport
  Sinal_B : Outport  Port=2
  Sinal_C : Outport  Port=3
  wires:
  Subsystem2/1(Out1) -> Sinal_C/1
  Subsystem1/1(Out1) -> Sinal_B/1
  Subsystem/1(Out1) -> Sinal_A/1
  Demux/1 -> Subsystem/1(In1)
  Demux/2 -> Subsystem/2(Input)
  Demux1/1 -> Subsystem1/1(In1)
  Demux1/2 -> Subsystem1/2(Input1)
  Demux2/1 -> Subsystem2/1(In1)
  Demux2/2 -> Subsystem2/2(Input2)
  Phasor_A/1 -> Demux/1
  Phasor_B/1 -> Demux1/1
  Phasor_C/1 -> Demux2/1

== system basic_cosimulation_c_1_sm_master/SM_Master/Circuit_ITM_Source_DP_AW/DP --> EMT ==
  Mag : Inport
  Phase : Inport  Port=2
  Compare To Constant : simulink/Logic and Bit Operations/Compare To Constant  relop=>=  const=2*pi  OutDataTypeStr=boolean
  Constant2 : Constant  Value=2*pi*60
  Integrator : Integrator  ExternalReset=rising  WrapState=on  WrappedStateUpperValue=2*pi  WrappedStateLowerValue=0  ShowStatePort=on
  Product4 : Product
  Sin3 : Trigonometry
  Sum4 : Sum  Inputs=|++
  I_injected : Outport
  wires:
  Product4/1 -> I_injected/1
  Mag/1 -> Product4/1
  Integrator/1 -> Sum4/2
  Phase/1 -> Sum4/1
  Sum4/1 -> Sin3/1
  Sin3/1 -> Product4/2
  Compare To Constant/1 -> Integrator/2
  Integrator/State -> Compare To Constant/1
  Constant2/1 -> Integrator/1

== system basic_cosimulation_c_1_sm_master/SM_Master/Circuit_ITM_Source_DP_AW/Dynamic Phasor coeficientes extraction ==
  EMT_Signal : Inport
  Demux : Demux  Outputs=3
  Fourier_A : spsFourierLib/Fourier  Freq=60  n=1  InInit=[1,0]  Ts=Ts
      settings: SourceProductBaseCode=PS
  Fourier_B : spsFourierLib/Fourier  Freq=60  n=1  InInit=[1,-120 ]  Ts=Ts
      settings: SourceProductBaseCode=PS
  Fourier_C : spsFourierLib/Fourier  Freq=60  n=1  InInit=[1,+120 ]  Ts=Ts
      settings: SourceProductBaseCode=PS
  Mux : Mux  Inputs=2
  Mux1 : Mux  Inputs=2
  Mux2 : Mux  Inputs=2
  deg->rad : Gain  Gain=pi/180  SaturateOnIntegerOverflow=on  OutDataTypeStr=Inherit: Same as input  ParamDataTypeStr=Inherit: Same as input
  deg->rad1 : Gain  Gain=pi/180  SaturateOnIntegerOverflow=on  OutDataTypeStr=Inherit: Same as input  ParamDataTypeStr=Inherit: Same as input
  deg->rad2 : Gain  Gain=pi/180  SaturateOnIntegerOverflow=on  OutDataTypeStr=Inherit: Same as input  ParamDataTypeStr=Inherit: Same as input
  Phasor_A : Outport
  Phasor_B : Outport  Port=2
  Phasor_C : Outport  Port=3
  wires:
  Demux/2 -> Fourier_B/1
  deg->rad1/1 -> Mux2/2
  Demux/3 -> Fourier_C/1
  Demux/1 -> Fourier_A/1
  Fourier_C/1 -> Mux1/1
  EMT_Signal/1 -> Demux/1
  Fourier_B/2 -> deg->rad1/1
  deg->rad2/1 -> Mux1/2
  Fourier_A/2 -> deg->rad/1
  Fourier_C/2 -> deg->rad2/1
  Fourier_A/1 -> Mux/1
  deg->rad/1 -> Mux/2
  Fourier_B/1 -> Mux2/1
  Mux/1 -> Phasor_A/1
  Mux2/1 -> Phasor_B/1
  Mux1/1 -> Phasor_C/1

== system basic_cosimulation_c_1_sm_master/SM_Master/Circuit_ITM_Source_DP_AW/Dynamic Phasor coeficients extraction ==
  EMT Signal : Inport
  Fourier_A : powerlib_meascontrol/Measurements/Fourier  Freq=60  n=1  InInit=[1,0]  Ts=Ts
  deg->rad : Gain  Gain=pi/180  SaturateOnIntegerOverflow=on  OutDataTypeStr=Inherit: Same as input  ParamDataTypeStr=Inherit: Same as input
  Mag : Outport
  Phase : Outport  Port=2
  wires:
  deg->rad/1 -> Phase/1
  Fourier_A/2 -> deg->rad/1
  Fourier_A/1 -> Mag/1
  EMT Signal/1 -> Fourier_A/1

== system basic_cosimulation_c_1_sm_master/SM_Master/Circuit_ITM_Source_DP_AW/Subsystem ==
  g : Inport
  Ideal Switch : spsIdealSwitchLib/Ideal Switch  Ron=0.001  Lon=0  IC=0  Rs=inf  Cs=0  Measurements=off
  Ideal Switch1 : spsIdealSwitchLib/Ideal Switch  Ron=0.001  Lon=0  IC=0  Rs=inf  Cs=0  Measurements=off
  Ideal Switch2 : spsIdealSwitchLib/Ideal Switch  Ron=0.001  Lon=0  IC=0  Rs=inf  Cs=0  Measurements=off
  2 : PMIOPort  Side=Right
  1 : PMIOPort  Port=2  Side=Right
  3 : PMIOPort  Port=3  Side=Right
  4 : PMIOPort  Port=4  Side=Left
  5 : PMIOPort  Port=5  Side=Left
  6 : PMIOPort  Port=6  Side=Left
  wires:
  g/1 -> Ideal Switch2/1, Ideal Switch1/1, Ideal Switch/1
  connections:
  Ideal Switch/LConn1 -- 4/RConn1
  Ideal Switch1/RConn1 -- 1/RConn1
  Ideal Switch2/RConn1 -- 3/RConn1
  5/RConn1 -- Ideal Switch1/LConn1
  6/RConn1 -- Ideal Switch2/LConn1
  Ideal Switch/RConn1 -- 2/RConn1

== system basic_cosimulation_c_1_sm_master/SM_Master/Circuit_ITM_Source_DP_AW/Three-Phase Controlled Y-Connected Current Source ==
  Ia : Inport
  Ib : Inport  Port=2
  Ic : Inport  Port=3
  Controlled Current Source : spsControlledCurrentSourceLib/Controlled Current Source  Initialize=on  Source_Type=AC  Amplitude=0  Phase=0  Frequency=0  Measurements=None
  Controlled Current Source1 : spsControlledCurrentSourceLib/Controlled Current Source  Initialize=on  Source_Type=AC  Amplitude=0  Phase=0  Frequency=0  Measurements=None
  Controlled Current Source2 : spsControlledCurrentSourceLib/Controlled Current Source  Initialize=on  Source_Type=AC  Amplitude=0  Phase=0  Frequency=0  Measurements=None
  Ground1 : spsGroundLib/Ground  LConnTagsString=a
  A : PMIOPort  Side=Left
  B : PMIOPort  Port=2  Side=Left
  C : PMIOPort  Port=3  Side=Left
  wires:
  Ia/1 -> Controlled Current Source/1
  Ic/1 -> Controlled Current Source2/1
  Ib/1 -> Controlled Current Source1/1
  connections:
  Controlled Current Source/RConn1 -- Controlled Current Source2/RConn1 -- Ground1/LConn1 -- Controlled Current Source1/RConn1
  C/RConn1 -- Controlled Current Source2/LConn1
  B/RConn1 -- Controlled Current Source1/LConn1
  Controlled Current Source/LConn1 -- A/RConn1

== system basic_cosimulation_c_1_sm_master/SM_Master/Circuit_ITM_Source_DP_SFA/Controllable Voltage Source  ==
  Amplitude [V] : Inport
  Phase [Deg] : Inport  Port=2
  Frequency [Hz] : Inport  Port=3
  Constant1 : Constant  Value=2*pi/3
  Controlled Voltage Source3 : spsControlledVoltageSourceLib/Controlled Voltage Source  Initialize=on  Source_Type=AC  Amplitude=0  Phase=0  Frequency=0  Measurements=None
  Controlled Voltage Source4 : spsControlledVoltageSourceLib/Controlled Voltage Source  Initialize=on  Source_Type=AC  Amplitude=0  Phase=0  Frequency=0  Measurements=None
  Controlled Voltage Source5 : spsControlledVoltageSourceLib/Controlled Voltage Source  Initialize=on  Source_Type=AC  Amplitude=0  Phase=0  Frequency=0  Measurements=None
  Cos : Trigonometry  Operator=cos
  Cos1 : Trigonometry  Operator=cos
  Cos2 : Trigonometry  Operator=cos
  Gain : Gain  Gain=2*pi
  Gain1 : Gain  Gain=pi/180
  Ground5 : spsGroundLib/Ground  LConnTagsString=a
  Integrator : Integrator  WrappedStateUpperValue=2*pi  WrappedStateLowerValue=0
  Product : Product
  Product1 : Product
  Product2 : Product
  Scope : Scope
  Sum : Sum  Inputs=++-
  Sum1 : Sum  Inputs=+++
  Sum2 : Sum  Inputs=|++
  A : PMIOPort  Side=Right
  B : PMIOPort  Port=2  Side=Right
  C : PMIOPort  Port=3  Side=Right
  wires:
  Sum/1 -> Cos1/1
  Amplitude [V]/1 -> Product2/1, Product1/1, Product/1
  Integrator/1 -> Scope/1, [phase]
  Gain/1 -> Integrator/1
  Phase [Deg]/1 -> Gain1/1
  Constant1/1 -> Sum/3, Sum1/2
  Sum2/1 -> Cos/1
  Product/1 -> Controlled Voltage Source3/1
  Cos/1 -> Product/2
  [phase] -> Sum2/1, Sum/2, Sum1/1
  Product1/1 -> Controlled Voltage Source4/1
  Product2/1 -> Controlled Voltage Source5/1
  Sum1/1 -> Cos2/1
  Cos1/1 -> Product1/2
  Cos2/1 -> Product2/2
  Frequency [Hz]/1 -> [freq_ref], Gain/1
  Gain1/1 -> Sum1/3, Sum/1, Sum2/2
  connections:
  Controlled Voltage Source4/RConn1 -- B/RConn1
  Controlled Voltage Source3/RConn1 -- A/RConn1
  Controlled Voltage Source5/RConn1 -- C/RConn1
  Controlled Voltage Source4/LConn1 -- Ground5/LConn1 -- Controlled Voltage Source5/LConn1 -- Controlled Voltage Source3/LConn1

== system basic_cosimulation_c_1_sm_master/SM_Master/Circuit_ITM_Source_DP_SFA/DP --> EMT ==
  Mag : Inport
  Phase : Inport  Port=2
  Compare To Constant : simulink/Logic and Bit Operations/Compare To Constant  relop=>=  const=2*pi  OutDataTypeStr=boolean
  Constant2 : Constant  Value=2*pi*60
  Integrator : Integrator  ExternalReset=rising  WrapState=on  WrappedStateUpperValue=2*pi  WrappedStateLowerValue=0  ShowStatePort=on
  Product4 : Product
  Sin3 : Trigonometry
  Sum4 : Sum  Inputs=|++
  I_injected : Outport
  wires:
  Product4/1 -> I_injected/1
  Mag/1 -> Product4/1
  Integrator/1 -> Sum4/2
  Phase/1 -> Sum4/1
  Sum4/1 -> Sin3/1
  Sin3/1 -> Product4/2
  Compare To Constant/1 -> Integrator/2
  Integrator/State -> Compare To Constant/1
  Constant2/1 -> Integrator/1

== system basic_cosimulation_c_1_sm_master/SM_Master/Circuit_ITM_Source_DP_SFA/Dynamic Phasor coeficients extraction ==
  EMT Signal : Inport
  Fourier_A : powerlib_meascontrol/Measurements/Fourier  Freq=60  n=1  InInit=[1,0]  Ts=Ts
  deg->rad : Gain  Gain=pi/180  SaturateOnIntegerOverflow=on  OutDataTypeStr=Inherit: Same as input  ParamDataTypeStr=Inherit: Same as input
  Mag : Outport
  Phase : Outport  Port=2
  wires:
  deg->rad/1 -> Phase/1
  Fourier_A/2 -> deg->rad/1
  Fourier_A/1 -> Mag/1
  EMT Signal/1 -> Fourier_A/1

== system basic_cosimulation_c_1_sm_master/SM_Master/Circuit_ITM_Source_DP_SFA/Phasor_to_Time_Domain_SFA ==
  Dynamic_Phasor : Inport
  Complex to Real-Imag4 : ComplexToRealImag
  Constant : Constant  Value=offset
  Demux : Demux  Outputs=3
  Demux1 : Demux  Outputs=2
  Gain : Gain  Gain=pi/180
  Gain3 : Gain  Gain=2*pi
  Gain4 : Gain  Gain=j*1
  Integrator : Integrator
  Magnitude-Angle to Complex : MagnitudeAngleToComplex
  Math Function : Math  SaturateOnIntegerOverflow=on
  Product : Product
  Real-Imag to Complex : RealImagToComplex
  Terminator : Terminator
  A : Outport
  B : Outport  Port=2
  C : Outport  Port=3
  wires:
  Demux/2 -> B/1
  Math Function/1 -> Product/2
  Gain4/1 -> Math Function/1
  Constant/1 -> Gain3/1
  Integrator/1 -> Gain4/1
  Dynamic_Phasor/1 -> Demux1/1
  Demux/1 -> A/1
  Product/1 -> Complex to Real-Imag4/1
  Gain3/1 -> Integrator/1
  Demux/3 -> C/1
  Complex to Real-Imag4/2 -> Terminator/1
  Complex to Real-Imag4/1 -> Demux/1
  Demux1/1 -> Real-Imag to Complex/1, Magnitude-Angle to Complex/1
  Demux1/2 -> Real-Imag to Complex/2, Gain/1
  Gain/1 -> Magnitude-Angle to Complex/2
  Real-Imag to Complex/1 -> Product/1

== system basic_cosimulation_c_1_sm_master/SM_Master/Circuit_ITM_Source_DP_SFA/Three-Phase Controlled Y-Connected Current Source ==
  Ia : Inport
  Ib : Inport  Port=2
  Ic : Inport  Port=3
  Controlled Current Source : spsControlledCurrentSourceLib/Controlled Current Source  Initialize=on  Source_Type=AC  Amplitude=0  Phase=0  Frequency=0  Measurements=None
  Controlled Current Source1 : spsControlledCurrentSourceLib/Controlled Current Source  Initialize=on  Source_Type=AC  Amplitude=0  Phase=0  Frequency=0  Measurements=None
  Controlled Current Source2 : spsControlledCurrentSourceLib/Controlled Current Source  Initialize=on  Source_Type=AC  Amplitude=0  Phase=0  Frequency=0  Measurements=None
  Ground1 : spsGroundLib/Ground  LConnTagsString=a
  A : PMIOPort  Side=Left
  B : PMIOPort  Port=2  Side=Left
  C : PMIOPort  Port=3  Side=Left
  wires:
  Ia/1 -> Controlled Current Source/1
  Ic/1 -> Controlled Current Source2/1
  Ib/1 -> Controlled Current Source1/1
  connections:
  Controlled Current Source/RConn1 -- Controlled Current Source2/RConn1 -- Ground1/LConn1 -- Controlled Current Source1/RConn1
  C/RConn1 -- Controlled Current Source2/LConn1
  B/RConn1 -- Controlled Current Source1/LConn1
  Controlled Current Source/LConn1 -- A/RConn1

== system basic_cosimulation_c_1_sm_master/SM_Master/Circuit_ITM_Source_DP_SFA/Time_Domain_To_Phasor_SFA ==
  EMT : Inport
  Complex to Magnitude-Angle : ComplexToMagnitudeAngle
  Complex to Magnitude-Angle1 : ComplexToMagnitudeAngle  Commented=on
  Complex to Real-Imag : ComplexToRealImag  Commented=on
  Complex to Real-Imag1 : ComplexToRealImag
  Constant : Constant  Value=offset
  Gain : Gain  Gain=j*(1/sqrt(3))*[0 1 -1; -1 0 1; 1 -1 0]  Multiplication=Matrix(K*u)
  Gain1 : Gain  Gain=180/pi
  Gain2 : Gain  Commented=on  Gain=j*(1/sqrt(3))*[0 1 -1; -1 0 1; 1 -1 0]  Multiplication=Matrix(K*u)
  Gain3 : Gain  Gain=-2*pi
  Gain4 : Gain  Gain=j*1
  Gain5 : Gain  Commented=on  Gain=180/pi
  Integrator : Integrator
  Math Function : Math  SaturateOnIntegerOverflow=on
  Mux1 : Mux  Inputs=2
  Mux2 : Mux  Commented=on  Inputs=2
  Mux3 : Mux  Inputs=2
  Phase/ Frequency Offset7 : commrflib2/Phase// Frequency Offset  Commented=on  phaseOffset=0  freqPort=off  freqOffset=-60
  Product : Product
  Scope : Scope
  Scope1 : Scope
  Scope2 : Scope  Commented=on  NumInputPorts=2
  Scope3 : Scope  Commented=on
  Scope4 : Scope  Commented=on
  Scope5 : Scope  Commented=on  NumInputPorts=2
  Scope6 : Scope
  Sum1 : Sum  Inputs=+|+
  Sum2 : Sum  Commented=on  Inputs=|++
  Dynamic_Phasor : Outport
  wires:
  Gain3/1 -> Integrator/1
  Sum1/1 -> Product/1
  Constant/1 -> Gain3/1
  Complex to Magnitude-Angle/1 -> Scope1/1, Mux1/1
  Gain/1 -> Sum1/1
  Gain1/1 -> Scope/1, Mux1/2
  Integrator/1 -> Gain4/1
  Math Function/1 -> Product/2
  Product/1 -> Complex to Real-Imag1/1, Complex to Magnitude-Angle/1
  Gain4/1 -> Math Function/1
  Complex to Magnitude-Angle/2 -> Gain1/1
  Gain2/1 -> Sum2/1
  Sum2/1 -> Scope2/2, Phase/ Frequency Offset7/1
  EMT/1 -> Sum1/2, Gain/1, Sum2/2, Scope2/1, Gain2/1
  Complex to Magnitude-Angle1/2 -> Gain5/1
  Phase/ Frequency Offset7/1 -> Complex to Real-Imag/1, Complex to Magnitude-Angle1/1
  Complex to Magnitude-Angle1/1 -> Scope4/1, Mux2/1
  Gain5/1 -> Scope3/1, Mux2/2
  Mux2/1 -> ?
  Complex to Real-Imag/2 -> Scope5/2
  Complex to Real-Imag/1 -> Scope5/1
  Complex to Real-Imag1/1 -> Mux3/1
  Complex to Real-Imag1/2 -> Mux3/2
  Mux3/1 -> Dynamic_Phasor/1, Scope6/1

== system basic_cosimulation_c_1_sm_master/SM_Master/OpComm/busStruct ==
  In1 : Inport
  In2 : Inport  Port=2
  Sub1 : Subsystem
  Sub2 : Subsystem
  Out1 : Outport
  Out2 : Outport  Port=2
  wires:
  Sub2/1(out) -> Out2/1
  In2/1 -> Sub2/1(in)
  Sub1/1(out) -> Out1/1
  In1/1 -> Sub1/1(in)
